simulink model "Verifica_EIG_20022026"  (R2025b)
settings: Solver=VariableStepAuto  StartTime=0.0  StopTime=10.0  RelTol=1e-3
values from neighbouring files (symbols this model uses):
  A = double(subs(A_sym, p_eq_instabile, val_instabili))    [SvolgimentoEsame.m]
  B = double(subs(B_sym, p_eq_instabile, val_instabili))    [SvolgimentoEsame.m]
undefined symbols (not defined in the file or in its folder): C_tot, D_tot, K_EIG, X0
settings Model: Creator=salvo  LastModifiedBy=salvo

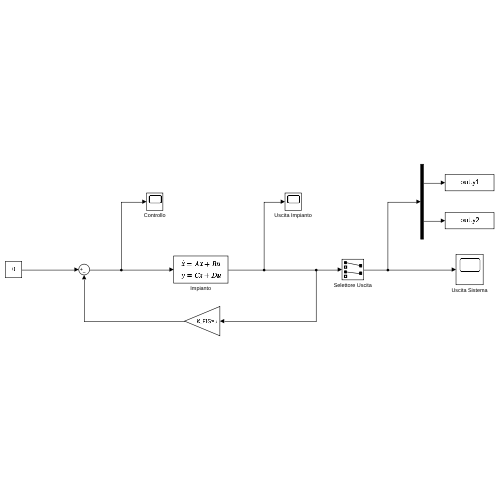
[thumbnail: Simulink's stored preview of the top-level diagram]
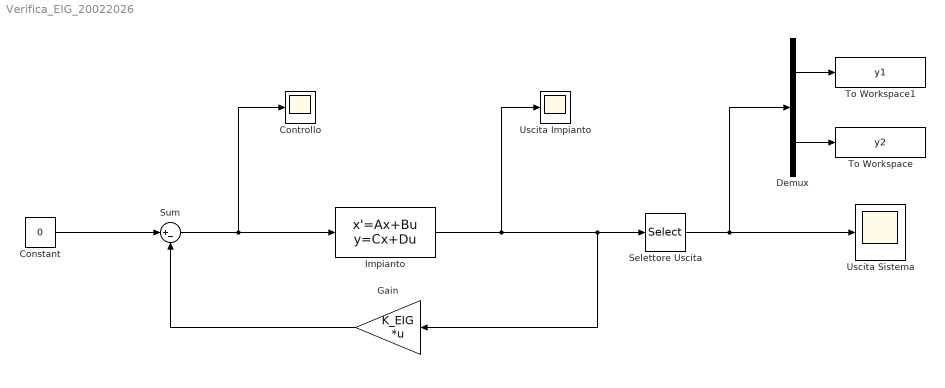
== system Verifica_EIG_20022026 ==
  Constant : Constant  Value=0
  Controllo : Scope
  Demux : Demux  Outputs=2
  Gain : Gain  Gain=K_EIG  Multiplication=Matrix(K*u)
  Impianto : StateSpace  A=A  B=B  C=C_tot  D=D_tot  InitialCondition=X0
  Selettore Uscita : Selector  InputPortWidth=4  IndexOptions=Index vector (dialog)  Indices=[1 3]  OutputSizes=1
  Sum : Sum  Inputs=|+-
  To Workspace : ToWorkspace  VariableName=y2  SaveFormat=Timeseries  SampleTime=-1
  To Workspace1 : ToWorkspace  VariableName=y1  SaveFormat=Timeseries  SampleTime=-1
  Uscita Impianto : Scope
      settings: DataLoggingVariableName=ScopeData2
  Uscita Sistema : Scope
      settings: ActiveDisplayYMinimum=-0.45879953771644416  ActiveDisplayYMaximum=1.2102734942238393
  wires:
  Constant/1 -> Sum/1
  Sum/1 -> Controllo/1, Impianto/1
  Impianto/1 -> Gain/1, Selettore Uscita/1, Uscita Impianto/1
  Gain/1 -> Sum/2
  Selettore Uscita/1 -> Demux/1, Uscita Sistema/1
  Demux/1 -> To Workspace1/1
  Demux/2 -> To Workspace/1
